simulink model "Landing_Check_1"  (R2023a)
settings: Solver=FixedStepAuto  StartTime=0.0  StopTime=0.  FixedStep=1.0  RelTol=1e-3
settings Model: Creator=horty  LastModifiedBy=horty
settings DataIOCC: SignalLogging=off  DSMLogging=off  SaveTime=off  ReturnWorkspaceOutputs=off

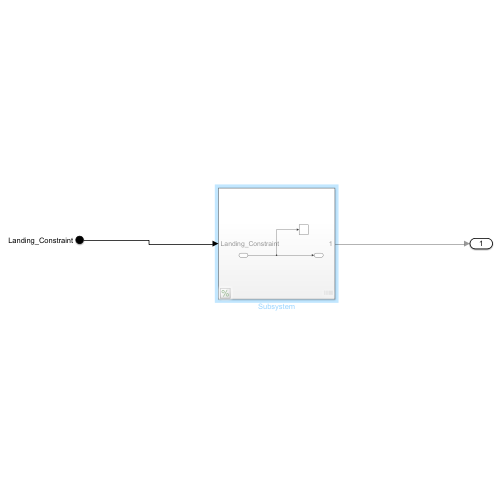
[thumbnail: Simulink's stored preview of the top-level diagram]
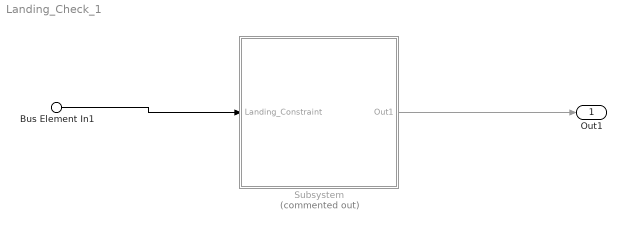
== system Landing_Check_1 ==
  Bus Element In1 : Inport  PortName=Landing_Constraint
  Subsystem : Subsystem  Commented=on
  Out1 : Outport
  wires:
  Bus Element In1/1 -> Subsystem/1(Landing_Constraint)
  Subsystem/1(Out1) -> Out1/1

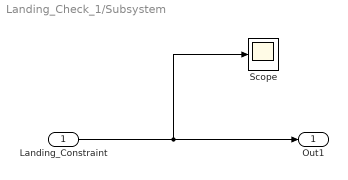
== system Landing_Check_1/Subsystem ==
  Landing_Constraint : Inport
  Scope : Scope
  Out1 : Outport
  wires:
  Landing_Constraint/1 -> Scope/1, Out1/1
